simulink subsystem "battery_module"  (R2021a)
settings: Solver=VariableStepAuto  StartTime=0.0  StopTime=10.0  RelTol=1e-3
settings Model: Creator=Carlo Edoardo  LastModifiedBy=miche

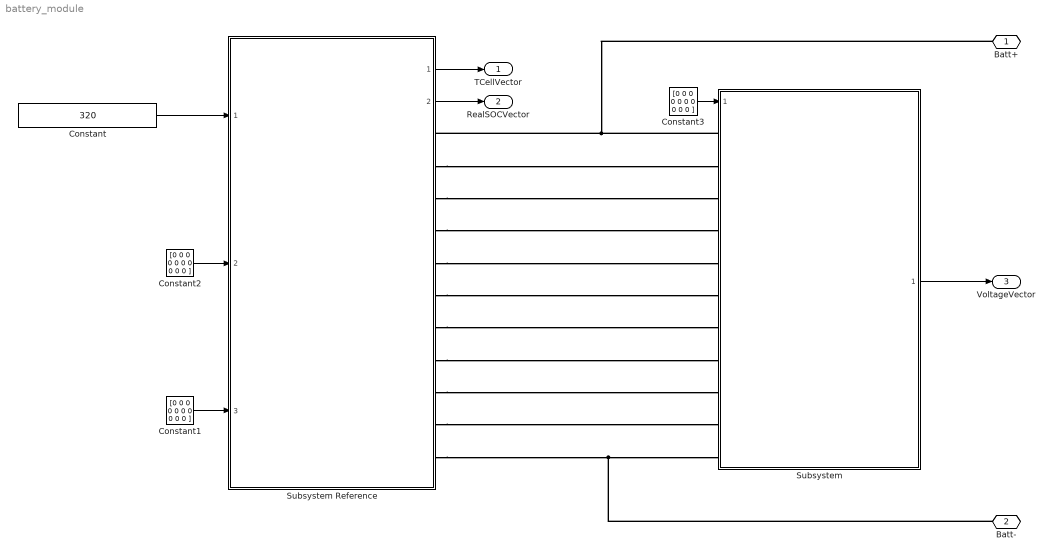
== system battery_module ==
  Constant : Constant  Value=320
  Constant1 : Constant  Value=[0 0 0 0 0 0 0 0 0 0 ]
  Constant2 : Constant  Value=[0 0 0 0 0 0 0 0 0 0 ]
  Constant3 : Constant  Value=[0 0 0 0 0 0 0 0 0 0 ]
  Subsystem : Subsystem  ReferencedSubsystem=balancing_passive
  Subsystem Reference : Subsystem  ReferencedSubsystem=battery_segment
  Batt+ : PMIOPort  Side=Right
  Batt- : PMIOPort  Port=2  Side=Right
  TCellVector : Outport
  RealSOCVector : Outport  Port=2
  VoltageVector : Outport  Port=3
  wires:
  Constant/1 -> Subsystem Reference/1
  Constant1/1 -> Subsystem Reference/3
  Constant2/1 -> Subsystem Reference/2
  Constant3/1 -> Subsystem/1
  Subsystem Reference/1 -> TCellVector/1
  Subsystem Reference/2 -> RealSOCVector/1
  Subsystem/1 -> VoltageVector/1
  connections:
  Batt+/RConn1 -- Subsystem Reference/RConn1 -- Subsystem/LConn1
  Subsystem Reference/RConn11 -- Subsystem/LConn11 -- Batt-/RConn1
  Subsystem Reference/RConn2 -- Subsystem/LConn2
  Subsystem Reference/RConn3 -- Subsystem/LConn3
  Subsystem Reference/RConn4 -- Subsystem/LConn4
  Subsystem Reference/RConn5 -- Subsystem/LConn5
  Subsystem Reference/RConn6 -- Subsystem/LConn6
  Subsystem Reference/RConn7 -- Subsystem/LConn7
  Subsystem Reference/RConn8 -- Subsystem/LConn8
  Subsystem Reference/RConn9 -- Subsystem/LConn9
  Subsystem Reference/RConn10 -- Subsystem/LConn10
